simulink model "dz21"  (R2023a)
settings: Solver=VariableStepAuto  StartTime=0.0  StopTime=10  RelTol=1e-3
values from neighbouring files (symbols this model uses):
  Cm = 1.3    [dz21 (3).m]    (also in dz21.m)
  Cw = 3.15    [dz21 (3).m]    (also in dz21.m)
  J = 7 * power(10, -6)    [dz21 (3).m]    (also in dz21.m)
  Ln = 0.0015    [dz21 (3).m]    (also in dz21.m)
  Lob = 0.013    [dz21 (3).m]    (also in dz21.m)
  Ra = 8    [dz21 (3).m]    (also in dz21.m)
settings Model: Creator=Андрей  LastModifiedBy=Андрей

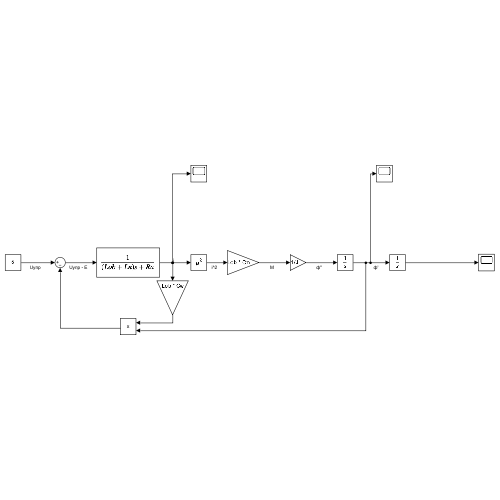
[thumbnail: Simulink's stored preview of the top-level diagram]
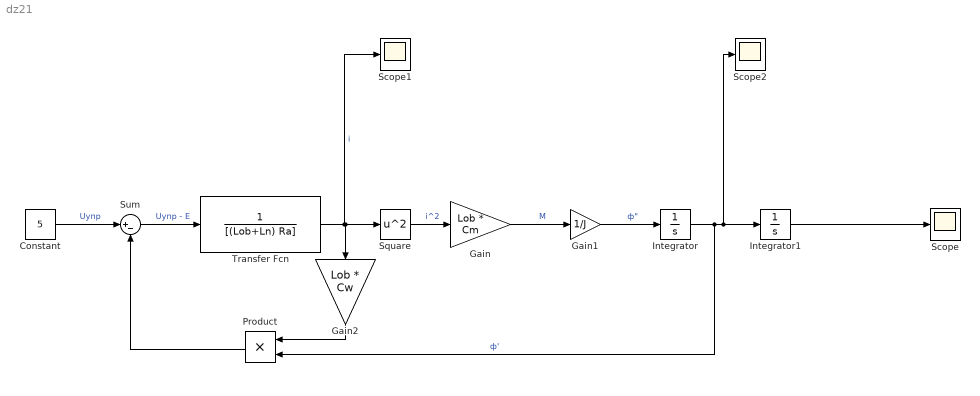
== system dz21 ==
  Constant : Constant  Value=5
  Gain : Gain  Gain=Lob * Cm
  Gain1 : Gain  Gain=1/J
  Gain2 : Gain  Gain=Lob * Cw
  Integrator : Integrator
  Integrator1 : Integrator
  Product : Product
  Scope : Scope
  Scope1 : Scope
  Scope2 : Scope
  Square : Math  Operator=square
  Sum : Sum  Inputs=|+-
  Transfer Fcn : TransferFcn  Denominator=[(Lob+Ln) Ra]
  wires:
  Constant/1 -> Sum/1  "Uупр"
  Sum/1 -> Transfer Fcn/1  "Uупр - E"
  Transfer Fcn/1 -> Gain2/1, Square/1, Scope1/1  "i"
  Square/1 -> Gain/1  "i^2"
  Gain/1 -> Gain1/1  "M"
  Gain1/1 -> Integrator/1  "ф\""
  Integrator/1 -> Product/2, Scope2/1, Integrator1/1  "ф'"
  Integrator1/1 -> Scope/1
  Gain2/1 -> Product/1
  Product/1 -> Sum/2
